simulink model "neptune_IDFT"  (R2023a)
settings: Solver=VariableStepAuto  StartTime=0.0  StopTime=10  RelTol=1e-3
undefined symbols (not defined in the file or in its folder): Radix
libraries: commseqgen3 x1, commdigbbndam3 x1, dspxfrm3 x1
settings Model: Creator=abraxas3d  LastModifiedBy=abraxas3d

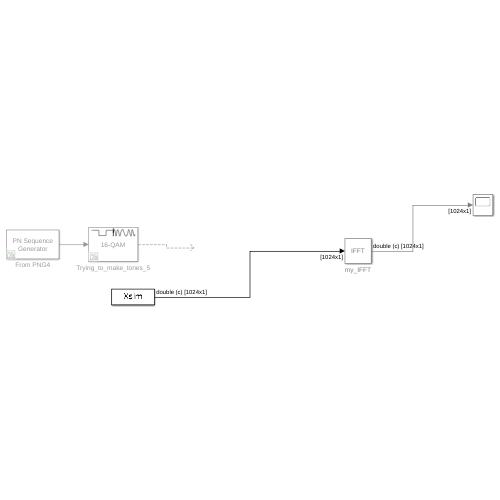
[thumbnail: Simulink's stored preview of the top-level diagram]
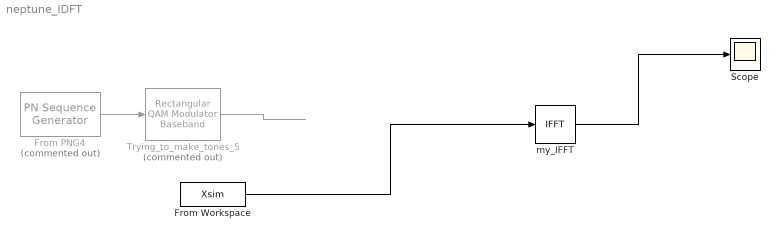
== system neptune_IDFT ==
  From Workspace : FromWorkspace  VariableName=Xsim
  From PNG4 : commseqgen3/PN Sequence Generator  Commented=on  poly='z^4 + z + 1'  ini_sta=[0 0 0 1]  outBitMaskSource=Dialog parameter  shift=0  outVarSiz=off  maxOutSizeMode=Dialog parameter  maxOutSize=[10 1]  Ts=1  sampPerFrame=1  reset=off  bitPackedOutputs=on  outDataType=Smallest unsigned integer  numPackedBits=4  bitPackDataSigned=off  bitPackedOutDType=Smallest integer
      settings: LibrarySourceBlock=|
      | commhdlsource/PN Sequence
      | Generator
  Scope : Scope
  Trying_to_make_tones_5 : commdigbbndam3/Rectangular QAM Modulator Baseband  Commented=on  M=16  InType=Integer  Enc=Gray  Mapping=[0:15]  PowType=Min. distance between symbols  MinDist=2  AvgPow=1  PeakPow=1  Ph=0  outDtype=Fixed-point  outWordLen=16  outUDDataType=sfix(16)  outFracLenMode=User-defined  outFracLen=0  outDataTypeStr=fixdt(1,16,0)  outLastDataTypeStr=fixdt(1,16,0)
      settings: LibrarySourceBlock=|
      | commhdldigbbndam/Rectangular QAM
      | Modulator
      | Baseband
  my_IFFT : dspxfrm3/IFFT  FFTImplementation=Radix-2  CompMethod=Table lookup  TableOpt=NEW  TableOptActive=Speed  BitRevOrder=off  cs_in=off  Normalize=on  InheritFFTLength=off  FFTLength=1024  WrapInput=on  mode=Complex  outSamplingMode=Sample based  roundingMode=Floor  overflowMode=off  firstCoeffDataTypeStr=Inherit: Same word length as input  firstCoeffLastDataTypeStr=Inherit: Same word length as input  outputMin=[]  outputMax=[]
  wires:
  my_IFFT/1 -> Scope/1
  From PNG4/1 -> Trying_to_make_tones_5/1
  Trying_to_make_tones_5/1 -> ?
  From Workspace/1 -> my_IFFT/1
